simulink subsystem "ZCD"  (R2022b)
settings: Solver=VariableStepAuto  StartTime=0.0  StopTime=10.0  RelTol=1e-3
libraries: simulink x1
settings Model: Creator=MAAM  LastModifiedBy=MAAM

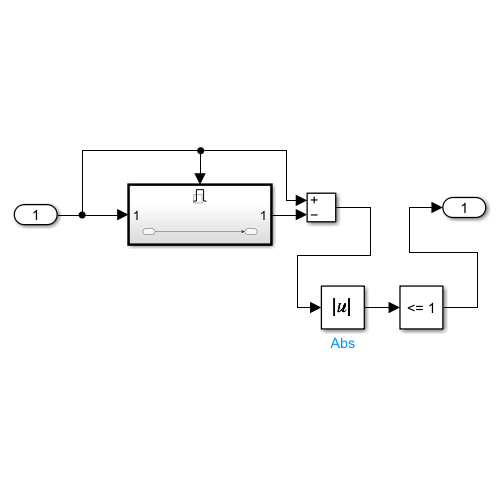
[thumbnail: Simulink's stored preview of the top-level diagram]
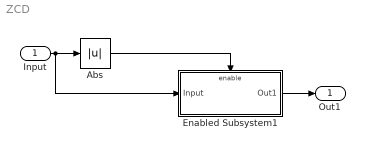
== system ZCD ==
  Input : Inport
  Abs : Abs  SaturateOnIntegerOverflow=off
  Enabled Subsystem1 : Subsystem  TreatAsAtomicUnit=on
  Out1 : Outport
  wires:
  Enabled Subsystem1/1(Out1) -> Out1/1
  Abs/1 -> Enabled Subsystem1/Enable
  Input/1 -> Abs/1, Enabled Subsystem1/1(Input)

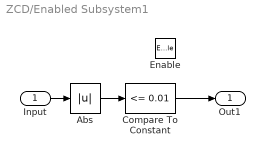
== system ZCD/Enabled Subsystem1 ==
  Input : Inport
  Enable : EnablePort  StatesWhenEnabling=reset
  Abs : Abs  SaturateOnIntegerOverflow=off
  Compare To Constant : simulink/Logic and Bit Operations/Compare To Constant  relop=<=  const=0.01  OutDataTypeStr=boolean
  Out1 : Outport
  wires:
  Input/1 -> Abs/1
  Abs/1 -> Compare To Constant/1
  Compare To Constant/1 -> Out1/1
